simulink model "linear_balan_bot_cont"  (R2018b)
settings: Solver=VariableStepAuto  StartTime=0.0  StopTime=10.0  MaxStep=0.001  RelTol=1e-3
undefined symbols (not defined in the file or in its folder): cart_d0, cart_d1, cart_d2, cart_d3, cart_d4, cart_n0, cart_n1, cart_n2, pend_d0, pend_d1, pend_d2, pend_d3, pend_n0, pend_n1
libraries: simulink x1
settings Model: Creator=Ikarus  LastModifiedBy=Ikarus

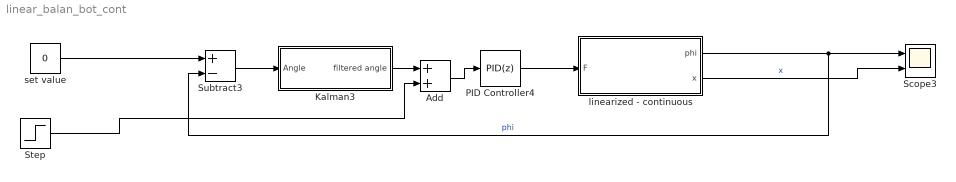
== system linear_balan_bot_cont ==
  Add : Sum
  Kalman3 : Subsystem  mask{step_time=0.01}
      mask prompts: step_time "step time"
  PID Controller4 : simulink/Continuous/PID Controller  Controller=PID  Form=Parallel  TimeDomain=Discrete-time  SampleTime=-1  IntegratorMethod=Forward Euler  FilterMethod=Forward Euler  ControllerParametersSource=internal  P=94.3174432822609  I=179.101520876593  D=7.29108455594587  UseFilter=on  N=1162.58764416015  TunerSelectOption=Transfer Function Based (PID Tuner App)  InitialConditionSource=internal  InitialConditionForIntegrator=0  InitialConditionForFilter=0  DifferentiatorICPrevScaledInput=0  ExternalReset=none  TrackingMode=off  Kt=1  LimitOutput=off  UpperSaturationLimit=inf  LowerSaturationLimit=-inf  LinearizeAsGain=on  AntiWindupMode=none  Kb=1  POutMin=[]  POutMax=[]  IOutMin=[]  IOutMax=[]  DOutMin=[]  DOutMax=[]  NOutMin=[]  NOutMax=[]  SumOutMin=[]  SumOutMax=[]  SaturationOutMin=[]  SaturationOutMax=[]  PParamMin=[]  PParamMax=[]  IParamMin=[]  IParamMax=[]  DParamMin=[]  DParamMax=[]  NParamMin=[]  NParamMax=[]  KbParamMin=[]  KbParamMax=[]  KtParamMin=[]  KtParamMax=[]  KbOutMin=[]  KbOutMax=[]  KtOutMin=[]  KtOutMax=[]  IntegratorOutMin=[]  IntegratorOutMax=[]  FilterOutMin=[]  FilterOutMax=[]  SumI1OutMin=[]  SumI1OutMax=[]  SumI2OutMin=[]  SumI2OutMax=[]  SumI3OutMin=[]  SumI3OutMax=[]  SumI4OutMin=[]  SumI4OutMax=[]  SumDOutMin=[]  SumDOutMax=[]  DifferentiatorOutMin=[]  DifferentiatorOutMax=[]  FilterDiffOutCoefMin=[]  FilterDiffOutCoefMax=[]  ReciprocalOutMin=[]  ReciprocalOutMax=[]  SumDenOutMin=[]  SumDenOutMax=[]  SumNumOutMin=[]  SumNumOutMax=[]  DivideOutMin=[]  DivideOutMax=[]  IntegratorContinuousStateAttributes=''  IntegratorStateMustResolveToSignalObject=off  IntegratorRTWStateStorageClass=Auto  FilterContinuousStateAttributes=''  FilterStateMustResolveToSignalObject=off  FilterRTWStateStorageClass=Auto  ParallelPVariant=InternalParameters  IdealPVariant=Disabled  IVariant=InternalParameters  DVariant=InternalParameters  IntegratorVariant=Discrete  SatVariant=Disabled  AWVariant=Passthrough  PCopyVariant=Disabled  TRVariant=Disabled  FdbkBlocksVariant=Forward  IdealPFdbkVariant=Disabled  SatFdbkVariant=Disabled  DerivativeFilterVariant=ForwardEulerFilter  NVariant=InternalParameters  NCopyVariant=Disabled  FilterICVariant=InternalICsFilter  IntegratorICVariant=InternalICs  ExternalResetVariant=Disabled  TRSumVariant=Passthrough  SumFdbkVariant=Disabled  SumVariant=Sum_PID
  Scope3 : Scope  NumInputPorts=2
  Step : Step  Before=5*pi/180  After=0  SampleTime=0
  Subtract3 : Sum  Inputs=+-
  linearized - continuous : Subsystem
  set value : Constant  Value=0  SampleTime=-1
  wires:
  linearized - continuous/1(phi) -> Subtract3/2, Scope3/1  "phi"
  Kalman3/1(filtered angle) -> Add/1
  PID Controller4/1 -> linearized - continuous/1(F)
  Subtract3/1 -> Kalman3/1("Angle ")
  linearized - continuous/2(x) -> Scope3/2  "x"
  set value/1 -> Subtract3/1
  Step/1 -> Add/2
  Add/1 -> PID Controller4/1

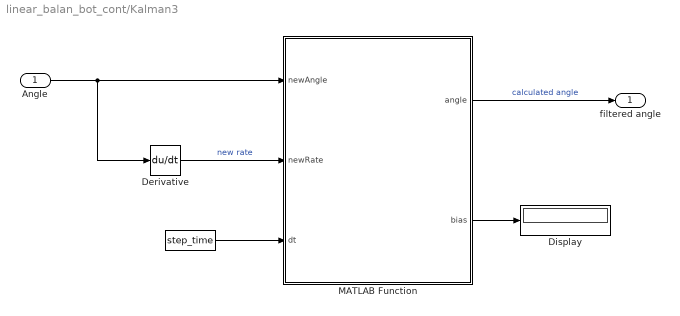
== system linear_balan_bot_cont/Kalman3 ==
  "Angle " : Inport
  "  " : Constant  Value=step_time
  Derivative : Derivative
  Display : Display
  MATLAB Function : MATLAB Function  TreatAsAtomicUnit=on
  filtered angle : Outport
  wires:
  "  "/1 -> MATLAB Function/3(dt)
  Derivative/1 -> MATLAB Function/2(newRate)  "new rate"
  MATLAB Function/1(angle) -> filtered angle/1  "calculated angle"
  "Angle "/1 -> Derivative/1, MATLAB Function/1(newAngle)
  MATLAB Function/2(bias) -> Display/1

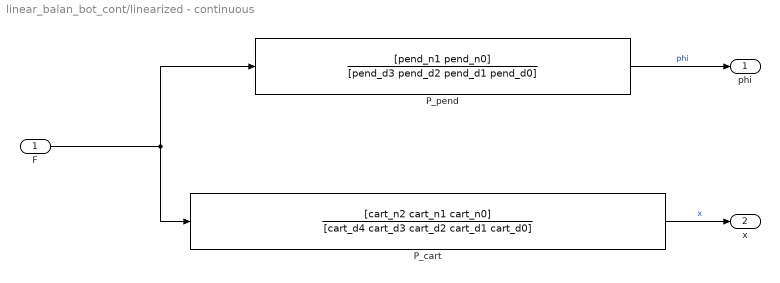
== system linear_balan_bot_cont/linearized - continuous ==
  F : Inport
  P_cart : TransferFcn  Numerator=[cart_n2 cart_n1 cart_n0]  Denominator=[cart_d4 cart_d3 cart_d2 cart_d1 cart_d0]
  P_pend : TransferFcn  Numerator=[pend_n1 pend_n0]  Denominator=[pend_d3 pend_d2 pend_d1 pend_d0]
  phi : Outport
  x : Outport  Port=2
  wires:
  P_cart/1 -> x/1  "x"
  F/1 -> P_pend/1, P_cart/1
  P_pend/1 -> phi/1  "phi"

== matlab function linear_balan_bot_cont/Kalman3/MATLAB Function ==
  settings: updateMethod=DISCRETE
  data: newAngle input; angle output; newRate input; dt input; bias output
function [angle,bias] = KalmanFil_Balanbot(newAngle,newRate,dt)
        % This script was adapted for its implementation in Simulink by R. Estrada (FH JOANNEUM 2017)
        % Based on KasBot V2  -  Kalman filter module - http:%www.x-firm.com/?page_id=145
        % Modified by Kristian Lauszus
        % More information: http:%blog.tkjelectronics.dk/2012/09/a-practical-approach-to-kalman-filter-and-how-to-implement-it

        % Discrete Kalman filter time update equations - Time Update ("Predict")
        % Update xhat - Project the state ahead
        
        coder.extrinsic('exist');
        
        % Declaration of persistent in memory variables (similar to declare global
        % variables)
   
        persistent init0 P K x;        
        
        % Initialization of typical sensor and noise variances 
        Q_angle = 0.001;
        Q_bias = 0.003; 
        R_measure = 0.03;
        
        % Declaration/initialization of main static matrices and vectors
        F = [1      -dt; 0      1];     % Transition matrix
        Q = [Q_angle  0; 0 Q_bias];     % Process noise covariance matrix  
        B = [dt ; 0];                   % Control-input model
        H = [1    0];                   % Observation model
        
        % SETUP: Executed only the first time      
        if isempty(init0)
            init0=0;
             % Declaration/initialization of main dynamic matrix and vectors
            P     = [0 0;0 0];  % Error covariance matrix
            K     = [0;0];      % Kalman gain vector
            x     = [0;0];      % State vector
        end

        % LOOP: Implementation of Kalman filter algorithm
        
        % Step 1 */          
        % Calculate prior state vector
        x = F * x + B * newRate;        

        % Step 2 */ 
        % Update estimation error covariance - Project the error covariance ahead               
         P = F * P * F' + Q * dt;  
                   
        % Step 3 */
        % Update estimate with measurement zk (newAngle)     
        y = newAngle - H * x;
        
        % Step 4 */
        % Discrete Kalman filter measurement update equations - Measurement Update ("Correct")              
        S = H * P * H' + R_measure;
        
        % Step 5 */
        % Compute the Kalman gain  
        K = P * H' / S;

        % Step 6 */
        % Update state vector
        x = x + K * y;
        
        % Step 7 */
        % Calculate estimation error covariance - Update the error covariance
        P = (eye(2) - K * H) * P;

        % RETURN: Update the function outputs
        angle = x(1);
        bias  = x(2);
